simulink model "boost_converter_2016a"  (Simulink 8.7)
settings: Solver=ode23t  SolverMode=SingleTasking  StartTime=0.0  StopTime=0.01  MaxStep=1e-7  RelTol=1e-3
libraries: powerlib x17
settings Model: Creator=sn  LastModifiedBy=sayan
settings DataIOCC: LimitDataPoints=off  SaveFormat=Dataset  ReturnWorkspaceOutputs=on
settings DebuggingCC: UnderspecifiedInitializationDetection=Simplified  MergeDetectMultiDrivingBlocksExec=error  SFUnexpectedBacktrackingDiag=error  SFNoUnconditionalDefaultTransitionDiag=error
settings HardwareCC: ProdBitPerPointer=64  ProdLargestAtomicFloat=Float  ProdIntDivRoundTo=Zero  ProdEndianess=LittleEndian  ProdWordSize=64  ProdHWDeviceType=Intel->x86-64 (Windows64)
settings ModelReferenceCC: PropagateSignalLabelsOutOfModel=on
settings SFSimCC: SimUseLocalCustomCode=on
settings RTWCC: RTWUseLocalCustomCode=on
settings GRTTargetCC: TargetLangStandard=C99 (ISO)  GeneratePreprocessorConditionals=Use local settings
settings ConfigComp: CovMetricSettings=dwe  CovHtmlReporting=off  CovSaveCumulativeToWorkspaceVar=off  CovSaveSingleToWorkspaceVar=off  CovModelRefEnable=off  CovExternalEMLEnable=on
settings SimscapeCC: SimscapeNormalizeSystem=off

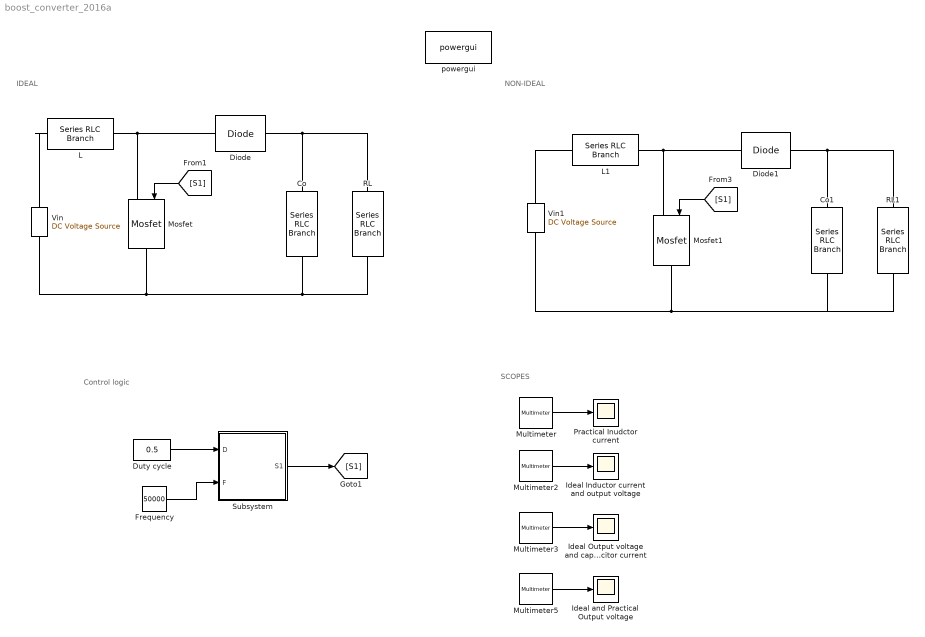
== system boost_converter_2016a ==
  note: Control logic
  note: SCOPES
  note: NON-IDEAL
  note: IDEAL
  Co : powerlib/Elements/Series RLC Branch  LConnTagsString=__new0  RConnTagsString=__new0  BranchType=C  Resistance=10e-3  Inductance=1e-3  SetiL0=off  InitialCurrent=0  Capacitance=54e-6  Setx0=off  InitialVoltage=0  Measurements=Branch voltage and current
  Co1 : powerlib/Elements/Series RLC Branch  LConnTagsString=__new0  RConnTagsString=__new0  BranchType=C  Resistance=10e-3  Inductance=1e-3  SetiL0=off  InitialCurrent=0  Capacitance=54e-6  Setx0=off  InitialVoltage=0  Measurements=Branch voltage and current
  Diode : powerlib/Power Electronics/Diode  Ron=1e-6  Lon=0  Vf=0  IC=0  UseSnubber=off  Rs=1e5  Cs=inf  Measurements=off
  Diode1 : powerlib/Power Electronics/Diode  Ron=1e-6  Lon=0  Vf=0  IC=0  UseSnubber=off  Rs=1e5  Cs=inf  Measurements=off
  Duty cycle : Constant  Value=0.5
  Frequency : Constant  Value=50000
  Ideal Inductor current and output voltage : Scope
  Ideal Output voltage and capacitor current : Scope
  Ideal and Practical Output voltage : Scope
  L : powerlib/Elements/Series RLC Branch  LConnTagsString=__new0  RConnTagsString=__new0  BranchType=L  Resistance=0.576  Inductance=115e-6  SetiL0=off  InitialCurrent=0  Capacitance=1e-6  Setx0=off  InitialVoltage=0  Measurements=Branch voltage and current
  L1 : powerlib/Elements/Series RLC Branch  LConnTagsString=__new0  RConnTagsString=__new0  BranchType=RL  Resistance=0.576  Inductance=115e-6  SetiL0=off  InitialCurrent=0  Capacitance=1e-6  Setx0=off  InitialVoltage=0  Measurements=Branch voltage and current
  Mosfet : powerlib/Power Electronics/Mosfet  Ron=1e-6  Lon=0  Rd=1e-6  Vfd=0  IC=0  Rs=1e5  Cs=inf  Measurements=off
  Mosfet1 : powerlib/Power Electronics/Mosfet  Ron=1e-6  Lon=0  Rd=1e-6  Vfd=0  IC=0  Rs=1e5  Cs=inf  Measurements=off
  Multimeter : powerlib/Measurements/Multimeter  PhasorSimulation=off  OutputType=Complex  sel=12  L=14  Gain=1  yselected={'Ib: L1'};  PSBOutputType=1  PSBequivalent=0  AxesSetting=[0,0.1,-100,100]  Display=0  SavedBlockNames=-11
  Multimeter2 : powerlib/Measurements/Multimeter  PhasorSimulation=off  OutputType=Complex  sel=[11 1]  L=14  Gain=[1 1]  yselected={'Ib: L','Ub: Co'};  PSBOutputType=1  PSBequivalent=0  AxesSetting=[0,0.1,-100,100]  Display=0  SavedBlockNames=-11
  Multimeter3 : powerlib/Measurements/Multimeter  PhasorSimulation=off  OutputType=Complex  sel=[1 9]  L=14  Gain=[1 1]  yselected={'Ub: Co','Ib: Co'};  PSBOutputType=1  PSBequivalent=0  AxesSetting=[0,0.1,-100,100]  Display=0  SavedBlockNames=-11
  Multimeter5 : powerlib/Measurements/Multimeter  PhasorSimulation=off  OutputType=Complex  sel=[1 2]  L=14  Gain=[1 1]  yselected={'Ub: Co','Ub: Co1'};  PSBOutputType=1  PSBequivalent=0  AxesSetting=[0,0.1,-100,100]  Display=0  SavedBlockNames=-11
  Practical Inudctor current : Scope
  RL : powerlib/Elements/Series RLC Branch  LConnTagsString=__new0  RConnTagsString=__new0  BranchType=R  Resistance=11.52  Inductance=1e-3  SetiL0=off  InitialCurrent=0  Capacitance=1e-6  Setx0=off  InitialVoltage=0  Measurements=Branch voltage and current
  RL1 : powerlib/Elements/Series RLC Branch  LConnTagsString=__new0  RConnTagsString=__new0  BranchType=R  Resistance=11.52  Inductance=1e-3  SetiL0=off  InitialCurrent=0  Capacitance=1e-6  Setx0=off  InitialVoltage=0  Measurements=Branch voltage and current
  Subsystem : Subsystem
  Vin : powerlib/Electrical Sources/DC Voltage Source  Amplitude=24  Measurements=Voltage
  Vin1 : powerlib/Electrical Sources/DC Voltage Source  Amplitude=24  Measurements=Voltage
  powergui : powerlib/powergui  Priority=1  SimulationMode=Discrete  SampleTime=1e-7  frequency=60  Iterations=50  frequencyindice=0  Pbase=100e6  ErrMax=1e-4  UnitsV=kV  UnitsW=MW  buscounter=0  FunctionMessages=off  echomessages=off  EnableUseOfTLC=off  CurrentSourceSwitches=on  DisableSnubberDevices=off  DisableRonSwitches=off  DisableVfSwitches=off  DisplayEquations=off  SolverType=Tustin/Backward Euler (TBE)  Interpol=off  ExternalGateDelay=off  methode=off  Ts=100  x0status=blocks  SPID=off  SwTol=0  HookPort=off  RestoreLinks=warning  ResistiveCurrentMeasurement=off  Frange=[0:2:500]  Ylog=off  Xlog=on  ShowGrid=off  save=off  variable=ZData  structure=0  ZoomFFT=off  StartTime=0.0  cycles=1  DisplayStyle=1  fundamental=60  FreqAxis=off  MaxFrequency=1000  frequencyindicesteady=1  RmsSteady=1  display=off
  wires:
  Duty cycle/1 -> Subsystem/1(D)
  Frequency/1 -> Subsystem/2(F)
  Subsystem/1(S1) -> [S1]
  [S1] -> Mosfet/1
  Multimeter/1 -> Practical Inudctor current/1
  Multimeter2/1 -> Ideal Inductor current and output voltage/1
  Multimeter3/1 -> Ideal Output voltage and capacitor current/1
  [S1] -> Mosfet1/1
  Multimeter5/1 -> Ideal and Practical Output voltage/1
  connections:
  L/LConn1 -- Vin/RConn1
  Mosfet/LConn1 -- Diode/LConn1 -- L/RConn1
  Mosfet/RConn1 -- RL/RConn1 -- Co/RConn1 -- Vin/LConn1
  Co/LConn1 -- RL/LConn1 -- Diode/RConn1
  Mosfet1/LConn1 -- Diode1/LConn1 -- L1/RConn1
  Mosfet1/RConn1 -- Co1/RConn1 -- RL1/RConn1 -- Vin1/LConn1
  Co1/LConn1 -- RL1/LConn1 -- Diode1/RConn1
  L1/LConn1 -- Vin1/RConn1

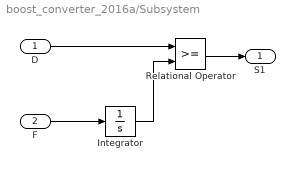
== system boost_converter_2016a/Subsystem ==
  D : Inport
  F : Inport  Port=2
  Integrator : Integrator  WrapState=on  WrappedStateUpperValue=1  WrappedStateLowerValue=0
  Relational Operator : RelationalOperator  OutDataTypeStr=boolean
  S1 : Outport
  wires:
  Integrator/1 -> Relational Operator/2
  F/1 -> Integrator/1
  D/1 -> Relational Operator/1
  Relational Operator/1 -> S1/1
